simulink model "lab2_1"  (R2015b)
settings: Solver=FixedStepDiscrete  StartTime=0.0  StopTime=inf  FixedStep=0.05  RelTol=1e-3
libraries: arduinolib x2
settings Model: SimulationMode=external  ExtModeTrigDuration=2  Creator=kando  LastModifiedBy=kando
settings OptimizationCC: OptimizeModelRefInitCode=on  LifeSpan=1  MaxStackSize=64
settings HardwareCC: ProdBitPerInt=16  ProdBitPerPointer=16  ProdLargestAtomicFloat=None  ProdWordSize=8  ProdHWDeviceType=Atmel->AVR
settings RTWCC: SystemTargetFile=ert.tlc  TemplateMakefile=ert_default_tmf  Description=Embedded Coder  Toolchain=Arduino AVR v1.6.1  BuildConfiguration=Faster Runs
settings CodeAppCC: IgnoreCustomStorageClasses=off
settings ERTTargetCC: SupportContinuousTime=on  SupportVariableSizeSignals=on

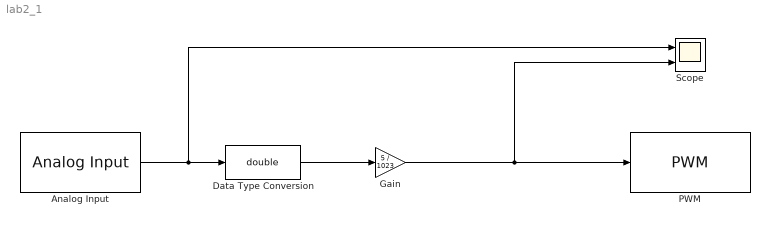
== system lab2_1 ==
  Analog Input : arduinolib/Analog Input  pinNumber=0  sampleTime=-1  blockPlatform=arduino
  Data Type Conversion : DataTypeConversion  OutDataTypeStr=double
  Gain : Gain  Gain=5 / 1023
      settings: AttributesFormatString=|
      | k.d2a:
      | %<Gain>
  PWM : arduinolib/PWM  pinNumber=13  blockPlatform=arduino
  Scope : Scope  NumInputPorts=2
  wires:
  Data Type Conversion/1 -> Gain/1
  Analog Input/1 -> Scope/1, Data Type Conversion/1
  Gain/1 -> Scope/2, PWM/1
